simulink model "trafficflow_tjunction_lights"  (R2021a)
settings: Solver=VariableStepAuto  StartTime=0.0  StopTime=10.0  RelTol=1e-3
settings Model: Creator=mariekutscher  LastModifiedBy=mariekutscher

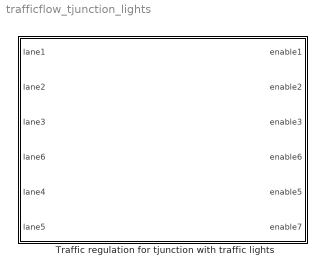
== system trafficflow_tjunction_lights ==
  Traffic regulation for tjunction with traffic lights : Stateflow chart  TreatAsAtomicUnit=on

== stateflow chart trafficflow_tjunction_lights/Traffic regulation for tjunction with traffic lights ==
  state Lane1_3_5
    entry: counter = 0;
    enable1 = 1;
    enable3 = 1;
    enable5 = 1;
    counter = counter + 1;
    exit: enable1 = 0; enable3 = 0; enable5 = 0;
  state Lane1_2_3
    entry: counter = 0;
    enable1 = 1;
    enable2 = 1;
    enable3 = 1;
    counter = counter + 1;
    exit: enable1 = 0; enable2 = 0; enable3 = 0;
  state Wait
    l1=lane1;
    l2=lane2;
    l3=lane3;
    l4=lane4;
    l5=lane5;
    l6=lane6;
  state Lane3_4_5
    entry: counter = 0;
    enable3 = 1;
    enable4 = 1;
    enable5 = 1;
    counter = counter + 1;
    exit: enable3 = 0; enable4 = 0; enable5 = 0;
  state Lane1_6
    entry: counter=0;
    enable1 = 1;
    enable6 = 1;
    counter = counter + 1;
    exit: enable1 = 0; enable6 = 0;
  Wait -> Lane1_3_5 [order 3] : [l1 == 1 || l3 == 1 | l5 == 1]
  Lane1_3_5 -> Wait : [counter > 5]{l1 = 0; l3 = 0; l5 = 0;}
  Wait -> Lane1_2_3 [order 1] : [l1 == 1|| l2 == 1 || l3 == 1]
  Lane1_2_3 -> Wait : [counter > 5]{l1 = 0; l2 = 0; l3 = 0;}
  (default) -> Wait
  Wait -> Lane3_4_5 [order 4] : [l3 == 1 || l4 == 1 || l5 == 1]
  Lane3_4_5 -> Wait : [counter > 5]{l3 = 0; l4 = 0; l5 = 0}
  Lane1_6 -> Wait : [counter > 5]{l1 = 0; l6 = 0;}
  Wait -> Lane1_6 [order 2] : [l1 == 1 || l6 == 1]
  data: lane1 input boolean size=1; lane2 input boolean size=1; lane3 input boolean size=1; enable1 output boolean size=1; enable2 output boolean size=1; enable3 output boolean size=1; lane6 input boolean size=1; enable6 output boolean size=1; lane4 input boolean size=1; lane5 input boolean size=1; enable5 output boolean size=1; enable7 output boolean size=1
